simulink model "CONT_CORE"  (Simulink 5.0)
settings: Solver=ode45  StartTime=0.0  StopTime=10.0  RelTol=1e-3
settings Model: LastModifiedBy=dsplab  BlockReductionOpt=off  BooleanDataType=off

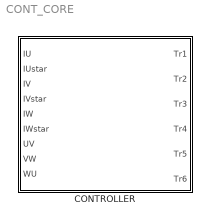
== system CONT_CORE ==
  CONTROLLER : Stateflow chart  TreatAsAtomicUnit=on

== stateflow chart CONTROLLER ==
  settings: updateMethod=CONTINUOUS  sampleTime=0.0001
  state A/
    state A1/
      during: Tr1=0;Tr3=0;Tr4=0;
      Tr2=0;Tr5=0;Tr6=0;
    state A2/
      during: Tr1=0; Tr3=0; Tr4=0; Tr2=0; Tr5=1;
      Tr6=1;
    (default) -> A1
  state B/
    state B1/
      during: Tr3=0;Tr5=0;Tr4=0;Tr2=0;
      Tr1=0; Tr6=0;
    state B2/
      during:Tr3=0;Tr5=0;Tr4=0;Tr2=0;
      Tr1=1; Tr6=1;
    (default) -> B1
  state C/
    state C1/
      during: Tr3=0;Tr5=0;Tr4=0;Tr2=0;
      Tr1=0; Tr6=0;
    state C2/
      during: Tr3=0;Tr5=0; Tr4=0; Tr6=0;
      Tr1=1; Tr2=1;
    (default) -> C1
  state D/
    state D1/
      during: Tr3=0;Tr5=0;Tr4=0;Tr2=0;
      Tr1=0; Tr6=0;
    state D2/
      during: Tr1=0; Tr5=0;Tr4=0; Tr6=0;
      Tr3=1; Tr2=1;
    (default) -> D1
  state E/
    state E1/
      during: Tr3=0;Tr5=0;Tr4=0;Tr2=0;
      Tr1=0; Tr6=0;
    state E2/
      during: Tr1=0; Tr5=0; Tr6=0; Tr2=0;
      Tr3=1; Tr4=1;
    (default) -> E1
  state F/
    state F1/
      during: Tr3=0;Tr5=0;Tr4=0;Tr2=0;
      Tr1=0; Tr6=0;
    state F2/
      during: Tr1=0; Tr3=0; Tr6=0; Tr2=0;
      Tr5=1; Tr4=1;
    (default) -> F1
  (default) -> A : [1]
  A1 -> A2 : [IV>IVstar]
  A2 -> A1 : [IV<IVstar]
  B1 -> B2 : [IU <IUstar]
  B2 -> B1 : [IU>IUstar]
  A -> B : [WU==1]
  C1 -> C2 : [IW>IWstar]
  C2 -> C1 : [IW<IWstar]
  B -> C : [VW==1]
  D1 -> D2 : [IV<IVstar]
  D2 -> D1 : [IV>IVstar]
  C -> D : [UV==1]
  E1 -> E2 : [IU>IUstar]
  E2 -> E1 : [IU<IUstar]
  D -> E : [WU==1]
  F1 -> F2 : [IW<IWstar]
  F2 -> F1 : [IU>IUstar]
  E -> F : [VW==1]
  F -> A : [UV==1]
  data: IU input double; IUstar input double; IV input double; IVstar input double; IW input double; IWstar input double; Tr1 output double; Tr2 output double; Tr3 output double; Tr4 output double; Tr5 output double; Tr6 output double; UV input double; VW input double; WU input double
